simulink model "Electric_Drives_Project"  (R2021b)
settings: Solver=VariableStepAuto  StartTime=0.0  StopTime=1  RelTol=1e-4
values from neighbouring files (symbols this model uses):
  Jr = 129*10^-7    (= 1.29e-05)    [Electric_Drives_Code.m]
  Kc = 71.3/1000    (= 0.0713)    [Electric_Drives_Code.m]
  La = 0.46/1000    (= 0.00046)    [Electric_Drives_Code.m]
  lts = 6.016*10^-5    (= 6.016e-05)    [Electric_Drives_Code.m]
  Ra = 1.72    [Electric_Drives_Code.m]
libraries: nesl_utility x13, ee_lib x11, fl_lib x10, simulink x3, spsTriangleGeneratorLib x1, spsStairGeneratorLib x1
settings Model: Creator=david  LastModifiedBy=david
settings SolverCC: ZeroCrossAlgorithm=Adaptive
settings DebuggingCC: IgnoredZcDiagnostic=none

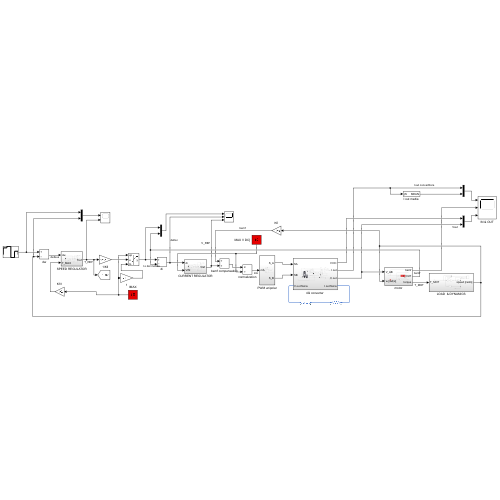
[thumbnail: Simulink's stored preview of the top-level diagram]
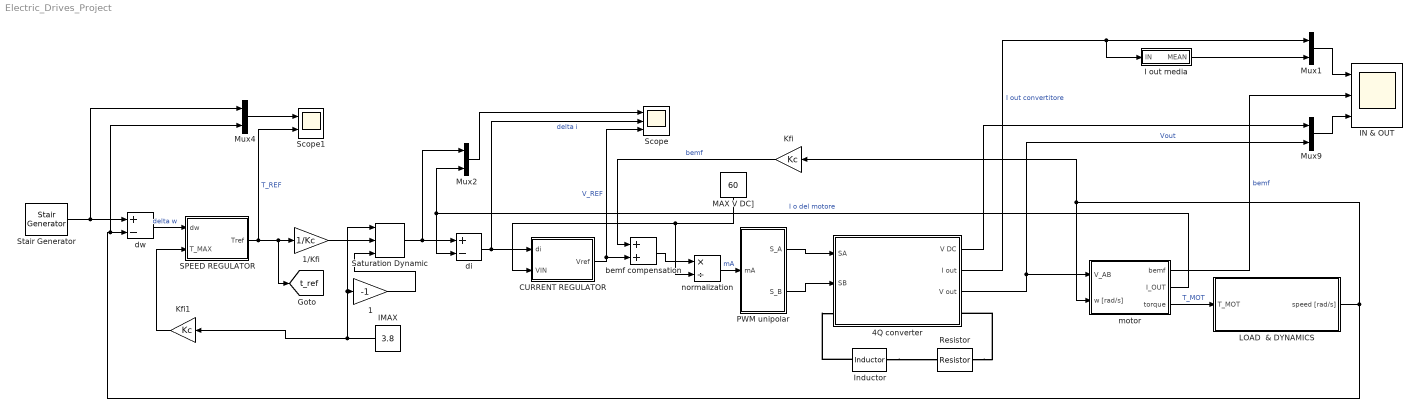
== system Electric_Drives_Project ==
  1 : Gain  Gain=-1
  1/Kfi : Gain  Gain=1/Kc
  "4Q converter " : Subsystem
  CURRENT REGULATOR : Subsystem
  "I out media " : Subsystem  mask{t_per=1/1000}
      mask prompts: t_per "period [s]"
  IMAX : Constant  Value=3.8
  IN & OUT : Scope  NumInputPorts=3
  Inductor : ee_lib/Passive/Inductor  l=1e-6 H  L_tol=20  enable_L_tol=0  tol_distribution=1  nSigma=4  r=0 Ohm  g=1e-9 1/Ohm  enable_operating_limits=0  operating_limit_action=2  max_working_current=1 A  power_rating=1 W  enable_faults=0  fault_action=1  lambdaPercent=50  k_faulted=0.9999  turnsShort=0  openCct=0  groundShort=0  groundShortG=0 1/Ohm  tau_fault=1e-3 s  enable_temporal_fault=0  t_fault=1 s  enable_behavioral_fault=0  max_permissible_voltage=100 V  n_fail_on_voltage=1  max_permissible_current=1 A  t_fail_on_current=1 s  i_L_specify=off  i_L_priority=High  i_L=0 A  i_L_nominal_specify=off  i_L_nominal_unit=A  i_L_nominal_value=1
  Kfi : Gain  Gain=Kc
  Kfi1 : Gain  Gain=Kc
  LOAD  & DYNAMICS : Subsystem
  MAX V DC] : Constant  Value=60
  Mux{1..2,4,9} (4 alike) : Mux  Inputs=2
  PWM unipolar : Subsystem
  Resistor : fl_lib/Electrical/Electrical Elements/Resistor  R=10 Ohm  i_specify=off  i_priority=None  i=0 A  i_nominal_specify=off  i_nominal_unit=A  i_nominal_value=1  v_specify=off  v_priority=None  v=0 V  v_nominal_specify=off  v_nominal_unit=V  v_nominal_value=1
  SPEED REGULATOR : Subsystem
  Saturation Dynamic : simulink/Discontinuities/Saturation Dynamic  OutMin=[]  OutMax=[]  OutDataTypeStr=Inherit: Same as second input  OutDataType=fixdt(1, 16)  OutScaling=2^-10  DoSatur=off
  Scope : Scope  NumInputPorts=3
  Scope1 : Scope  NumInputPorts=2
  Stair Generator : spsStairGeneratorLib/Stair Generator  t=[0, 0.2, 0.4, 0.6, 0.8, 1]  e=[0, 608, 760, -300, 300, 0]  Ts=0
  bemf compensation : Sum
  di : Sum  Inputs=+-
  dw : Sum  Inputs=+-
  motor : Subsystem
  normalization : Product  Inputs=*/
  tag scope: t_ref=global
  wires:
  SPEED REGULATOR/1(Tref) -> Scope1/2, [t_ref], 1/Kfi/1  "T_REF"
  1/1 -> Saturation Dynamic/3
  IMAX/1 -> Kfi1/1, 1/1, Saturation Dynamic/1
  normalization/1 -> PWM unipolar/1(mA)  "mA"
  LOAD  & DYNAMICS/1(speed [rad/s]) -> Mux4/2, dw/2, Kfi/1, motor/2(w [rad/s])
  "4Q converter "/2(I out) -> "I out media "/1(IN), Mux1/1  "I out convertitore"
  motor/2(I_OUT) -> di/2, Mux2/2  "I o del motore"
  1/Kfi/1 -> Saturation Dynamic/2
  motor/3(torque) -> LOAD  & DYNAMICS/1(T_MOT)  "T_MOT"
  Mux4/1 -> Scope1/1
  MAX V DC]/1 -> CURRENT REGULATOR/2(VIN), normalization/2
  Kfi1/1 -> SPEED REGULATOR/2(T_MAX)
  Mux1/1 -> IN & OUT/1
  dw/1 -> SPEED REGULATOR/1(dw)  "delta w"
  Kfi/1 -> bemf compensation/1  "bemf"
  Stair Generator/1 -> Mux4/1, dw/1
  CURRENT REGULATOR/1(Vref) -> Scope/3, bemf compensation/2  "V_REF"
  Saturation Dynamic/1 -> Mux2/1, di/1
  bemf compensation/1 -> normalization/1
  PWM unipolar/1(S_A) -> "4Q converter "/1(SA)
  Mux2/1 -> Scope/1
  di/1 -> Scope/2, CURRENT REGULATOR/1(di)  "delta i"
  PWM unipolar/2(S_B) -> "4Q converter "/2(SB)
  "4Q converter "/3(V out) -> Mux9/2, motor/1(V_AB)  "Vout"
  Mux9/1 -> IN & OUT/3
  "4Q converter "/1(V DC) -> Mux9/1
  "I out media "/1(MEAN) -> Mux1/2
  motor/1(bemf) -> IN & OUT/2  "bemf"
  connections:
  Resistor/LConn1 -- "4Q converter "/RConn1
  Inductor/LConn1 -- Resistor/RConn1
  Inductor/RConn1 -- "4Q converter "/LConn1

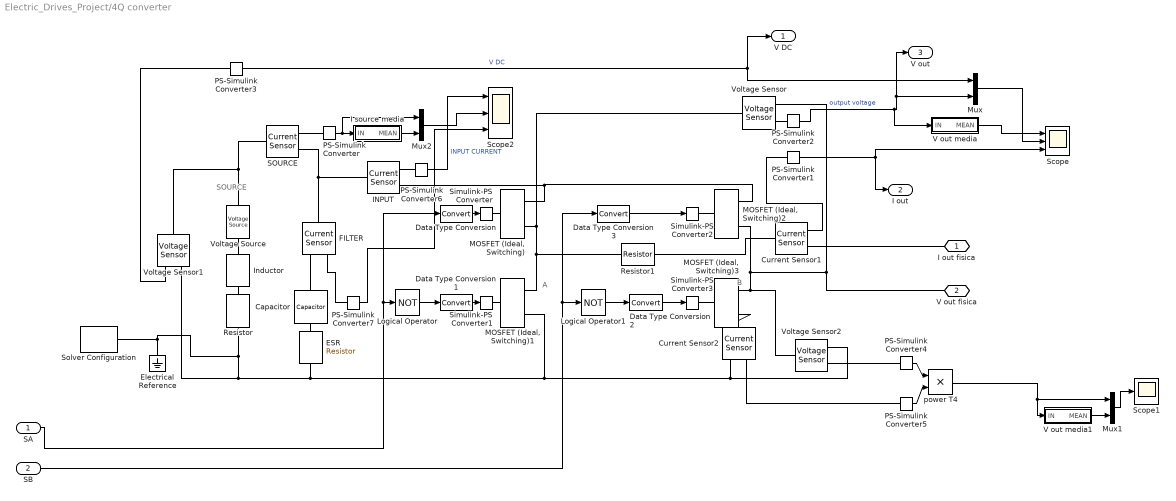
== system Electric_Drives_Project/4Q converter  ==
  note: B
  note: A
  note: SOURCE
  SA : Inport
  SB : Inport  Port=2
  Capacitor : ee_lib/Passive/Capacitor  cap_option=0  c=200e-3 F  Cvec=[1e-05, 1e-06] F  Vvec=[0, 10] V  CV_table_symmetry=1  f_vec=[1, 10] kHz  DFext_vec=[.8, 1.2]  C_tol=5  enable_C_tol=0  tol_distribution=1  nSigma=4  r=1e-6 Ohm  g=0 1/Ohm  averaging_period=0 s  enable_operating_limits=0  operating_limit_action=2  max_working_voltage_range=[-25, 25] V  power_rating=1 W  enable_faults=0  fault_action=1  Cscale_faulted=100  R_faulted=1e-3 Ohm  G_faulted=0 1/Ohm  tau_fault=1e-3 s  enable_temporal_fault=0  t_fault=1 s  enable_behavioral_fault=0  max_permissible_voltage_range=[-100, 100] V  t_fail_on_voltage=1 s  i_specify=off  i_priority=None  i=0 A  i_nominal_specify=off  i_nominal_unit=A  i_nominal_value=1  v_specify=off  v_priority=None  v=0 V  v_nominal_specify=off  v_nominal_unit=V  v_nominal_value=1  vc_specify=off  vc_priority=High  vc=0 V  vc_nominal_specify=off  vc_nominal_unit=V  vc_nominal_value=1
  Current Sensor1 : fl_lib/Electrical/Electrical Sensors/Current Sensor
  Current Sensor2 : fl_lib/Electrical/Electrical Sensors/Current Sensor
  Data Type Conversion{,1..3} (4 alike) : DataTypeConversion
  ESR : ee_lib/Passive/Resistor  R=0.1 Ohm  R_tol=5  enable_R_tol=0  tol_distribution=1  nSigma=4  enable_operating_limits=0  operating_limit_action=2  max_working_voltage=100 V  power_rating=1 W  enable_faults=0  fault_action=1  R_faulted=inf Ohm  enable_temporal_fault=0  t_fault=1 s  enable_behavioral_fault=0  max_permissible_current=1 A  t_fail_on_current=1 s  noise_mode=0  sample_time=1e-3 s  repeatability=1  auto_seed=3499211588  user_seed=0  Tdevice=25 degC  power_derating_T1=70 degC  power_derating_T2=155 degC  operating_temperature_range_vec=[-50, 150] degC  alpha=3.93e-3 1/K  Tmeas=25 degC  thermal_mass=100 J/K  temperature_specify=off  temperature_priority=High  temperature=298.15 K  temperature_nominal_specify=off  temperature_nominal_unit=K  temperature_nominal_value=1
  Electrical Reference : fl_lib/Electrical/Electrical Elements/Electrical Reference
  FILTER : fl_lib/Electrical/Electrical Sensors/Current Sensor
  I source media : Subsystem  mask{t_per=1/1000}
      mask prompts: t_per "period [s]"
  INPUT : fl_lib/Electrical/Electrical Sensors/Current Sensor
  Inductor : ee_lib/Passive/Inductor  l=0.0006 H  L_tol=20  enable_L_tol=0  tol_distribution=1  nSigma=4  r=0 Ohm  g=0 1/Ohm  enable_operating_limits=0  operating_limit_action=2  max_working_current=1 A  power_rating=1 W  enable_faults=0  fault_action=1  lambdaPercent=50  k_faulted=0.9999  turnsShort=0  openCct=0  groundShort=0  groundShortG=0 1/Ohm  tau_fault=1e-3 s  enable_temporal_fault=0  t_fault=1 s  enable_behavioral_fault=0  max_permissible_voltage=100 V  n_fail_on_voltage=1  max_permissible_current=1 A  t_fail_on_current=1 s  i_L_specify=off  i_L_priority=High  i_L=0 A  i_L_nominal_specify=off  i_L_nominal_unit=A  i_L_nominal_value=1
  Logical Operator : Logic  Operator=NOT  AllPortsSameDT=off  OutDataTypeStr=boolean
  Logical Operator1 : Logic  Operator=NOT  AllPortsSameDT=off  OutDataTypeStr=boolean
  MOSFET (Ideal, Switching){,1..3} (4 alike) : ee_lib/Semiconductors & Converters/MOSFET (Ideal, Switching)  Rds=0.1 Ohm  Goff=1e-6 1/Ohm  Vth=0.5 V  diode_param=1  diode_Vf=0.8 V  diode_Ron=0.001 Ohm  diode_Goff=1e-5 1/Ohm  diode_C=50e-9 F  diode_iRM=-235 A  diode_iF=300 A  diode_idot=-50 A/us  diode_trr_param=1  diode_trr_factor=3  diode_trr=15 us  diode_Qrr=1500 s*uA  thermal_loss_option=ee.enum.converters.thermalLossOption.constantvalues  Von_data=[0, 1.1, 1.3, 1.45, 1.75, 2.25, 2.7; 0, 1, 1.15, 1.35, 1.7, 2.35, 3] V  Tj=[298.15, 398.15] K  Iout_data=[0, 10, 50, 100, 200, 400, 600] A  Eon_data=[0, .29, 1.43, 2.86, 5.71, 13.14, 22.86; 0, .57, 2.63, 5.14, 10.29, 20.57, 30.29] * 1e-3 J  Eoff_data=[0, .21, 1.07, 2.14, 4.29, 9.86, 17.14; 0, .43, 1.97, 3.86, 7.71, 15.43, 22.71] * 1e-3 J  Tj_loss=[298.15, 398.15] K  Iout_data_loss=[0, 10, 50, 100, 200, 400, 600] A  Eon_scalar=22.86e-3 J  Eoff_scalar=17.14e-3 J  Voff=300 V  Iout_scalar=600 A  diodeModelType=ee.enum.converters.diodeModelType.pwl  diodeTableType=ee.enum.diode.tableType.IfMat  diode_IfMat=[.07, .12, .19, 1.75, 4.24, 7.32, 11.2; .16, .3, .72, 2.14, 4.02, 6.35, 9.12] A  diode_VfMat=[.9, 1.15, 1.25, 1.5, 1.75, 2.17, 2.6, 2.85; .58, .68, .75, 1.1, 1.38, 1.77, 2.27, 2.7] V  diode_TjVec=[25, 125] degC  diode_VfVec=[.5, .7, .9, 1.3, 1.7, 2.1, 2.5] V  diode_IfVec=[.1, .2, .5, 1, 2, 4, 7, 10] A  diode_Vr=-600 V  diode_Ls=150 nH  diode_Erec=0.03 J  thermal_network_parameterization=ee.enum.thermalNetworkTopology.external  Rth=[.03, .2] K/W  Rth_Cauer=[.03, .1, .2] K/W  Rth_Foster=[.03, .2] K/W  thermal_mass_parameterization=ee.enum.thermalNetwork.timeconstant  thermal_mass=[3, 25] J/K  thermal_mass_Cauer=[3, 10, 25] J/K  thermal_mass_Foster=[33, 50] J/K  thermal_time_constant=[.1, 5] s  thermal_time_constant_Cauer=[.1, 1, 5] s  thermal_time_constant_Foster=[1, 10] s  thermal_mass_initial_temperatures=[25, 25] degC  thermal_mass_initial_temperatures_Cauer=[25, 25, 25] degC  junction_thermal_mass=0.1 J/K  steadyState_Foster=simscape.enum.onoff.on  Tvec_initial_Foster=[25, 25, 25, 25] degC  no_thermal_network=0  junction_temperature_specify=off  junction_temperature_priority=None  junction_temperature=25 degC  junction_temperature_nominal_specify=off  junction_temperature_nominal_unit=degC  junction_temperature_nominal_value=1  vT_specify=off  vT_priority=None  vT=0 V  vT_nominal_specify=off  vT_nominal_unit=V  vT_nominal_value=1  Qj_specify=off  Qj_priority=None  Qj=0 W  Qj_nominal_specify=off  Qj_nominal_unit=W  Qj_nominal_value=1
  Mux : Mux  Inputs=2
  Mux1 : Mux  Inputs=2
  Mux2 : Mux  Inputs=2
  PS-Simulink Converter{,1..7} (8 alike) : nesl_utility/PS-Simulink Converter  PhysicalDomain=network_engine_domain  SubClassName=ps_output  LeftPortType=input  RightPortType=output  PseudoPeriodic=off  Frequencies=[]  Unit=inherit  AffineConversion=off
      settings: SourceProductBaseCode=PW,SS
  Resistor : ee_lib/Passive/Resistor  R=0.6 Ohm  R_tol=5  enable_R_tol=2  tol_distribution=1  nSigma=4  enable_operating_limits=0  operating_limit_action=2  max_working_voltage=100 V  power_rating=1 W  enable_faults=0  fault_action=1  R_faulted=inf Ohm  enable_temporal_fault=0  t_fault=1 s  enable_behavioral_fault=0  max_permissible_current=1 A  t_fail_on_current=1 s  noise_mode=0  sample_time=1e-3 s  repeatability=1  auto_seed=3890346746  user_seed=0  Tdevice=25 degC  power_derating_T1=70 degC  power_derating_T2=155 degC  operating_temperature_range_vec=[-50, 150] degC  alpha=3.93e-3 1/K  Tmeas=25 degC  thermal_mass=100 J/K  temperature_specify=off  temperature_priority=High  temperature=298.15 K  temperature_nominal_specify=off  temperature_nominal_unit=K  temperature_nominal_value=1
  Resistor1 : ee_lib/Passive/Resistor  R=7 Ohm  R_tol=5  enable_R_tol=2  tol_distribution=1  nSigma=4  enable_operating_limits=0  operating_limit_action=2  max_working_voltage=100 V  power_rating=1 W  enable_faults=0  fault_action=1  R_faulted=inf Ohm  enable_temporal_fault=0  t_fault=1 s  enable_behavioral_fault=0  max_permissible_current=1 A  t_fail_on_current=1 s  noise_mode=0  sample_time=1e-3 s  repeatability=1  auto_seed=3037630589  user_seed=0  Tdevice=25 degC  power_derating_T1=70 degC  power_derating_T2=155 degC  operating_temperature_range_vec=[-50, 150] degC  alpha=3.93e-3 1/K  Tmeas=25 degC  thermal_mass=100 J/K  temperature_specify=off  temperature_priority=High  temperature=298.15 K  temperature_nominal_specify=off  temperature_nominal_unit=K  temperature_nominal_value=1
  SOURCE : fl_lib/Electrical/Electrical Sensors/Current Sensor
  Scope : Scope  NumInputPorts=3
  Scope1 : Scope
  Scope2 : Scope  NumInputPorts=3
  Simulink-PS Converter{,1..3} (4 alike) : nesl_utility/Simulink-PS Converter  PhysicalDomain=network_engine_domain  SubClassName=ps_input  LeftPortType=input  RightPortType=output  PseudoPeriodic=off  Frequencies=[]  NoiseDistribution=none  NoiseParameters=[]  Unit=1  AffineConversion=off  FilteringAndDerivatives=provide  SimscapeFilterOrder=1  InputFilterTimeConstant=0.001  UdotUserProvided=0
      settings: SourceProductBaseCode=PW,SS
  Solver Configuration : nesl_utility/Solver Configuration  PhysicalDomain=network_engine_domain  SubClassName=solver  LeftPortType=input  RightPortType=generic  Tones=[]  Harmonics=[]  SimulateNoise=off  Profile=off  UseLocalSampling=off  EnableSwitchedLinearOptims=on  FrequencyDomain=off  UseCCode=off  RelTol=0.001  AbsTol=1e-06  MinStep=1e-09  ToWorkspace=off  RevertToSquareIcSolve=off  NumHomotopyIterations=100  PhasorMode=off  PhasorModeNumHarmonics=1  DoDC=off  ResidualTolerance=1e-09  UseLocalSolver=off  LocalSolverChoice=NE_BACKWARD_EULER_ADVANCER  LocalSolverSampleTime=0.001  DoFixedCost=off  MaxNonlinIter=3  MaxModeIter=2  ComputeImpulses=off  ImpulseIterations=2  LinearAlgebra=auto  EquationFormulation=NE_TIME_EF  DelaysMemoryBudget=1024  AutomaticFiltering=on  FilteringTimeConstant=0.001  PartitionStorageMethod=AS_NEEDED  PartitionMemoryBudget=1024  PartitionMethod=ROBUST
      settings: SourceProductBaseCode=PW,SS
  V out media : Subsystem  mask{t_per=1/1000}
      mask prompts: t_per "period [s]"
  V out media1 : Subsystem  mask{t_per=1/1000}
      mask prompts: t_per "period [s]"
  Voltage Sensor : fl_lib/Electrical/Electrical Sensors/Voltage Sensor
  Voltage Sensor1 : fl_lib/Electrical/Electrical Sensors/Voltage Sensor
  Voltage Sensor2 : fl_lib/Electrical/Electrical Sensors/Voltage Sensor
  Voltage Source : ee_lib/Sources/Voltage Source  dc_voltage=60 V  ac_voltage=0 V  ac_shift=0 rad  ac_frequency=60 Hz  noise_mode=0  PSD=0 V^2/Hz  repeatability=1  auto_seed=545404223  user_seed=0  sample_time=1e-3 s  i_specify=off  i_priority=None  i=0 A  i_nominal_specify=off  i_nominal_unit=A  i_nominal_value=1  v_specify=off  v_priority=None  v=0 V  v_nominal_specify=off  v_nominal_unit=V  v_nominal_value=1
  power T4 : Product
  I out fisica : PMIOPort  Side=Right
  V out fisica : PMIOPort  Port=2  Side=Left
  V DC : Outport
  I out : Outport  Port=2
  V out : Outport  Port=3
  wires:
  Mux/1 -> Scope/2
  PS-Simulink Converter4/1 -> power T4/1
  Logical Operator/1 -> Data Type Conversion1/1
  PS-Simulink Converter7/1 -> Scope2/3
  power T4/1 -> Mux1/1, V out media1/1(IN)
  Mux2/1 -> Scope2/2
  PS-Simulink Converter3/1 -> V DC/1, Mux/1  "V DC"
  PS-Simulink Converter5/1 -> power T4/2
  Data Type Conversion3/1 -> Simulink-PS Converter2/1
  Data Type Conversion2/1 -> Simulink-PS Converter3/1
  Logical Operator1/1 -> Data Type Conversion2/1
  Data Type Conversion/1 -> Simulink-PS Converter/1
  SA/1 -> Logical Operator/1, Data Type Conversion/1
  PS-Simulink Converter2/1 -> V out media/1(IN), V out/1, Mux/2  "output voltage"
  Data Type Conversion1/1 -> Simulink-PS Converter1/1
  SB/1 -> Data Type Conversion3/1, Logical Operator1/1
  PS-Simulink Converter1/1 -> I out/1, Scope/3
  PS-Simulink Converter6/1 -> Scope2/1  "INPUT CURRENT"
  V out media/1(MEAN) -> Scope/1
  V out media1/1(MEAN) -> Mux1/2
  Mux1/1 -> Scope1/1
  I source media/1(MEAN) -> Mux2/2
  PS-Simulink Converter/1 -> Mux2/1, I source media/1(IN)
  connections:
  Voltage Sensor1/RConn2 -- Solver Configuration/RConn1 -- Electrical Reference/LConn1 -- Resistor/RConn1 -- "MOSFET (Ideal, Switching)1"/RConn2 -- Voltage Sensor2/RConn2 -- Current Sensor2/RConn2 -- ESR/RConn1
  INPUT/LConn1 -- SOURCE/RConn2 -- FILTER/LConn1
  "MOSFET (Ideal, Switching)3"/RConn1 -- "MOSFET (Ideal, Switching)2"/RConn2 -- V out fisica/RConn1 -- Voltage Sensor/RConn2 -- Voltage Sensor2/LConn1
  SOURCE/LConn1 -- Voltage Source/LConn1 -- Voltage Sensor1/LConn1
  "MOSFET (Ideal, Switching)"/RConn1 -- "MOSFET (Ideal, Switching)2"/RConn1 -- INPUT/RConn2
  Voltage Sensor/LConn1 -- "MOSFET (Ideal, Switching)"/RConn2 -- "MOSFET (Ideal, Switching)1"/RConn1 -- Resistor1/LConn1
  ESR/LConn1 -- Capacitor/RConn1
  "MOSFET (Ideal, Switching)3"/RConn2 -- Current Sensor2/LConn1
  Voltage Sensor2/RConn1 -- PS-Simulink Converter4/LConn1
  Inductor/LConn1 -- Voltage Source/RConn1
  "MOSFET (Ideal, Switching)3"/LConn1 -- Simulink-PS Converter3/RConn1
  Resistor/LConn1 -- Inductor/RConn1
  PS-Simulink Converter6/LConn1 -- INPUT/RConn1
  FILTER/RConn1 -- PS-Simulink Converter7/LConn1
  Current Sensor2/RConn1 -- PS-Simulink Converter5/LConn1
  Voltage Sensor/RConn1 -- PS-Simulink Converter2/LConn1
  "MOSFET (Ideal, Switching)2"/LConn1 -- Simulink-PS Converter2/RConn1
  SOURCE/RConn1 -- PS-Simulink Converter/LConn1
  Voltage Sensor1/RConn1 -- PS-Simulink Converter3/LConn1
  Simulink-PS Converter/RConn1 -- "MOSFET (Ideal, Switching)"/LConn1
  Simulink-PS Converter1/RConn1 -- "MOSFET (Ideal, Switching)1"/LConn1
  FILTER/RConn2 -- Capacitor/LConn1
  Current Sensor1/RConn2 -- I out fisica/RConn1
  Current Sensor1/RConn1 -- PS-Simulink Converter1/LConn1
  Resistor1/RConn1 -- Current Sensor1/LConn1

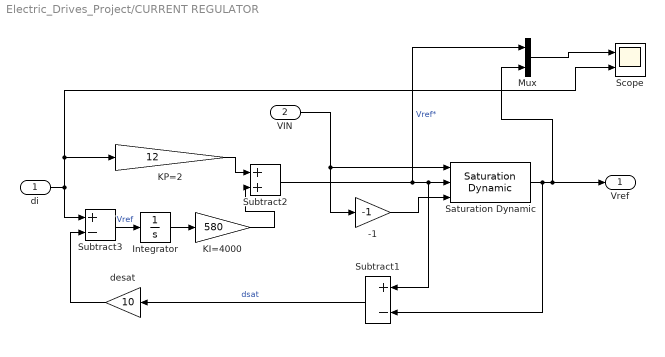
== system Electric_Drives_Project/CURRENT REGULATOR ==
  di : Inport
  VIN : Inport  Port=2
  -1 : Gain  Gain=-1
  Integrator : Integrator
  KI=4000 : Gain  Gain=580
  KP=2 : Gain  Gain=12
  Mux : Mux  Inputs=2
  Saturation Dynamic : simulink/Discontinuities/Saturation Dynamic  OutMin=[]  OutMax=[]  OutDataTypeStr=Inherit: Same as second input  OutDataType=fixdt(1, 16)  OutScaling=2^-10  DoSatur=off
  Scope : Scope  NumInputPorts=2
  Subtract1 : Sum  Inputs=+-
  Subtract2 : Sum
  Subtract3 : Sum  Inputs=+-
  desat : Gain  Gain=10
  Vref : Outport
  wires:
  Integrator/1 -> KI=4000/1
  di/1 -> Scope/2, KP=2/1, Subtract3/1
  KI=4000/1 -> Subtract2/2
  KP=2/1 -> Subtract2/1
  Subtract2/1 -> Mux/1, Subtract1/1, Saturation Dynamic/2  "Vref*"
  Saturation Dynamic/1 -> Subtract1/2, Mux/2, Vref/1
  VIN/1 -> -1/1, Saturation Dynamic/1
  -1/1 -> Saturation Dynamic/3
  Subtract1/1 -> desat/1  "dsat"
  desat/1 -> Subtract3/2
  Subtract3/1 -> Integrator/1  "Vref"
  Mux/1 -> Scope/1

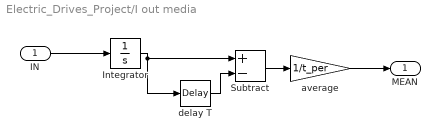
== system Electric_Drives_Project/I out media  ==
  IN : Inport
  Integrator : Integrator
  Subtract : Sum  Inputs=+-
  average : Gain  Gain=1/t_per
  delay T : TransportDelay  DelayTime=t_per  BufferSize=2048
  MEAN : Outport
  wires:
  delay T/1 -> Subtract/2
  Integrator/1 -> delay T/1, Subtract/1
  average/1 -> MEAN/1
  Subtract/1 -> average/1
  IN/1 -> Integrator/1

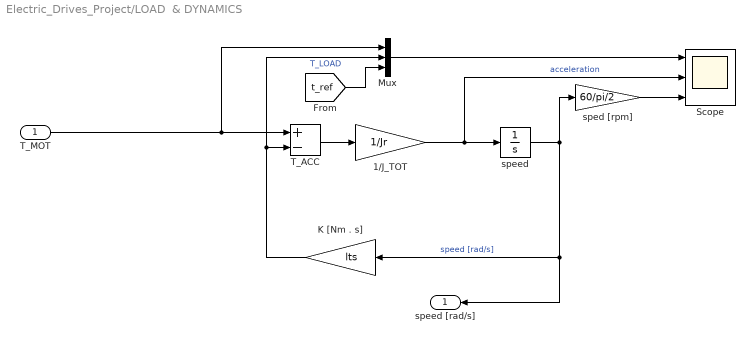
== system Electric_Drives_Project/LOAD  & DYNAMICS ==
  T_MOT : Inport
  1/J_TOT : Gain  Gain=1/Jr
  K [Nm . s] : Gain  Gain=lts
  Mux : Mux  Inputs=3
  Scope : Scope  NumInputPorts=3
  T_ACC : Sum  Inputs=+-
  sped [rpm] : Gain  Gain=60/pi/2
  speed : Integrator
  speed [rad/s] : Outport
  wires:
  K [Nm . s]/1 -> Mux/2, T_ACC/2  "T_LOAD"
  1/J_TOT/1 -> Scope/2, speed/1  "acceleration"
  T_ACC/1 -> 1/J_TOT/1
  T_MOT/1 -> Mux/1, T_ACC/1
  speed/1 -> sped [rpm]/1, K [Nm . s]/1, speed [rad/s]/1  "speed [rad/s]"
  Mux/1 -> Scope/1
  sped [rpm]/1 -> Scope/3
  [t_ref] -> Mux/3

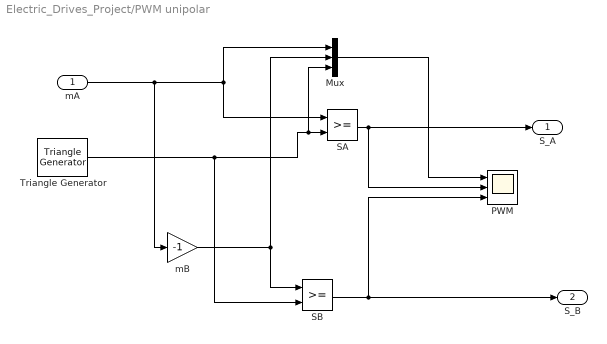
== system Electric_Drives_Project/PWM unipolar ==
  mA : Inport
  Mux : Mux  Inputs=3
  PWM : Scope  NumInputPorts=3
  SA : RelationalOperator  OutDataTypeStr=boolean  RndMeth=Simplest
  SB : RelationalOperator  OutDataTypeStr=boolean  RndMeth=Simplest
  Triangle Generator : spsTriangleGeneratorLib/Triangle Generator  Freq=5e4  Phase=90  Ts=0
  mB : Gain  Gain=-1
  S_A : Outport
  S_B : Outport  Port=2
  wires:
  Mux/1 -> PWM/1
  mB/1 -> Mux/2, SB/1
  Triangle Generator/1 -> Mux/3, SA/2, SB/2
  SB/1 -> S_B/1, PWM/3
  SA/1 -> S_A/1, PWM/2
  mA/1 -> mB/1, Mux/1, SA/1

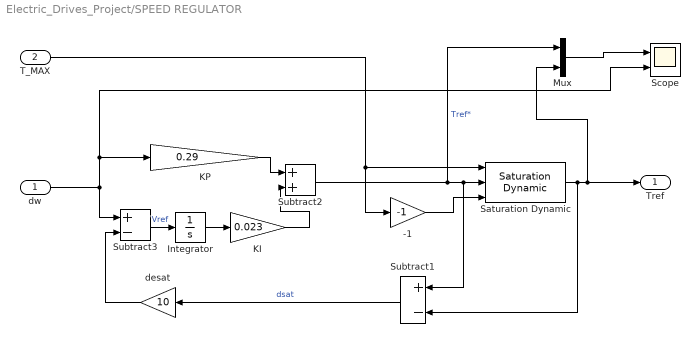
== system Electric_Drives_Project/SPEED REGULATOR ==
  dw : Inport
  T_MAX : Inport  Port=2
  -1 : Gain  Gain=-1
  Integrator : Integrator
  KI : Gain  Gain=0.023
  KP : Gain  Gain=0.29
  Mux : Mux  Inputs=2
  Saturation Dynamic : simulink/Discontinuities/Saturation Dynamic  OutMin=[]  OutMax=[]  OutDataTypeStr=Inherit: Same as second input  OutDataType=fixdt(1, 16)  OutScaling=2^-10  DoSatur=off
  Scope : Scope  NumInputPorts=2
  Subtract1 : Sum  Inputs=+-
  Subtract2 : Sum
  Subtract3 : Sum  Inputs=+-
  desat : Gain  Gain=10
  Tref : Outport
  wires:
  Mux/1 -> Scope/1
  Subtract3/1 -> Integrator/1  "Vref"
  desat/1 -> Subtract3/2
  Subtract1/1 -> desat/1  "dsat"
  -1/1 -> Saturation Dynamic/3
  T_MAX/1 -> Saturation Dynamic/1, -1/1
  Saturation Dynamic/1 -> Tref/1, Mux/2, Subtract1/2
  Subtract2/1 -> Saturation Dynamic/2, Subtract1/1, Mux/1  "Tref*"
  KP/1 -> Subtract2/1
  KI/1 -> Subtract2/2
  dw/1 -> Subtract3/1, KP/1, Scope/2
  Integrator/1 -> KI/1

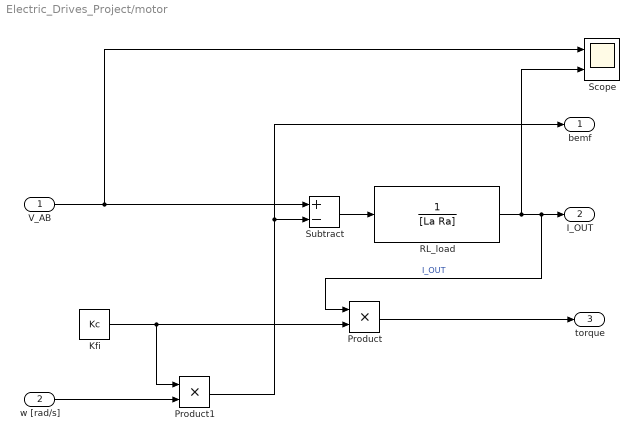
== system Electric_Drives_Project/motor ==
  V_AB : Inport
  w [rad/s] : Inport  Port=2
  Kfi : Constant  Value=Kc
  Product : Product
  Product1 : Product
  RL_load : TransferFcn  Denominator=[La Ra]
  Scope : Scope  NumInputPorts=2
  Subtract : Sum  Inputs=+-
  bemf : Outport
  I_OUT : Outport  Port=2
  torque : Outport  Port=3
  wires:
  Subtract/1 -> RL_load/1
  V_AB/1 -> Scope/1, Subtract/1
  RL_load/1 -> Scope/2, Product/1, I_OUT/1  "I_OUT"
  Product1/1 -> bemf/1, Subtract/2
  Kfi/1 -> Product1/1, Product/2
  Product/1 -> torque/1
  w [rad/s]/1 -> Product1/2

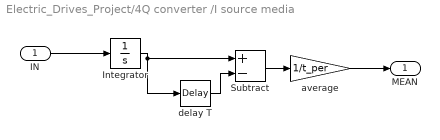
== system Electric_Drives_Project/4Q converter /I source media ==
  IN : Inport
  Integrator : Integrator
  Subtract : Sum  Inputs=+-
  average : Gain  Gain=1/t_per
  delay T : TransportDelay  DelayTime=t_per  BufferSize=2048
  MEAN : Outport
  wires:
  delay T/1 -> Subtract/2
  Integrator/1 -> delay T/1, Subtract/1
  average/1 -> MEAN/1
  Subtract/1 -> average/1
  IN/1 -> Integrator/1

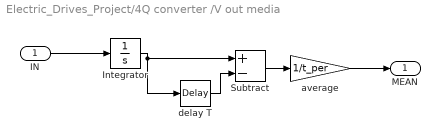
== system Electric_Drives_Project/4Q converter /V out media ==
  IN : Inport
  Integrator : Integrator
  Subtract : Sum  Inputs=+-
  average : Gain  Gain=1/t_per
  delay T : TransportDelay  DelayTime=t_per  BufferSize=2048
  MEAN : Outport
  wires:
  delay T/1 -> Subtract/2
  Integrator/1 -> delay T/1, Subtract/1
  average/1 -> MEAN/1
  Subtract/1 -> average/1
  IN/1 -> Integrator/1

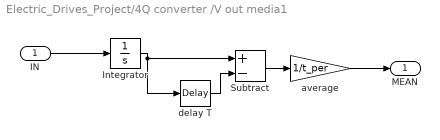
== system Electric_Drives_Project/4Q converter /V out media1 ==
  IN : Inport
  Integrator : Integrator
  Subtract : Sum  Inputs=+-
  average : Gain  Gain=1/t_per
  delay T : TransportDelay  DelayTime=t_per  BufferSize=2048
  MEAN : Outport
  wires:
  delay T/1 -> Subtract/2
  Integrator/1 -> delay T/1, Subtract/1
  average/1 -> MEAN/1
  Subtract/1 -> average/1
  IN/1 -> Integrator/1
